simulink model "E55_1030"  (R2019b)
settings: Solver=FixedStepDiscrete  StartTime=0.0  StopTime=10  FixedStep=0.0005  RelTol=1e-3  EnableMultiTasking=on
InitFcn:
  | ecucoder_canfd
  | load('DATA_Plimit.mat')
  | a=0.775;
  | b=0.775;
  | kf=-50000;
  | kr=-50000;
  | m=226+75;
  | Iz=100;
  | u=0.85;
  | g=9.8;
  | L=a+b;
  | xi=0.1;
  | r=0.226;
  | Lw=1.171;
  | Tm=21;
  | i=15.9;
  | Jw=0.504;
  | Pmax=20000;
  | mw=19.3;
  | mb=148.9+75;
  | hg=0.280;
model workspace (MAT data in the model file):
  Initial_Steer_Position = 0
values from neighbouring files (symbols this model uses):
  SOC = [2.5 5 7.5 10 20 30 40 50 60 70 80 90 ... (14 elements, 14x1)]    [DATA_Plimit.mat]
  SOC_Discharge = [2.04592350211 2.57821618825 3.10671863859 3.63118835861 4.15200192786 4.66837694959 5.18149950051 5.69046162564 6.19532286188 6.696400261 7.19347596839 7.68712157998 ... (473 elements, 1x473)]    [DATA_Plimit.mat]
  VOLTAGE = [459.1488 476.0844 485.9448 487.344 492.822 498.8016 503.382 509.1108 518.8128 531.2472 544.5132 558.4656 ... (14 elements, 14x1)]    [DATA_Plimit.mat]
undefined symbols (not defined in the file or in its folder): DiscIntNeverNeededParam, H, HALL10, HALL6, HALL7, HALL8, HALL9, HPWM1, HPWM3, I_AN05_5V, I_AN07_5V, I_AN08_5V, I_AN09_5V, I_AN10_5V, I_SW11_H, I_SW12_H, I_SW13_H, I_SW14_H, I_SW15_H, I_SW16_H, I_SW17_H, I_SW18_H, I_SW19_H, LS1A2, O_HS1A2, O_HS1A8
libraries: ec311lib x152, simulink x92, canmsglib x30, canfdmsglib x2
(part 6 of 6)

== system E55_1030/Function-Call Subsystem2/Triggered Subsystem/AMK_Setpoints_Motor3/AMK_TorqueLimitNegativ ==
  AMK_TorqueLimitNegativ : Inport
  AMK_TorqueLimitNegativABS : Abs
  AMK_TorqueLimitNegativCOV : DataTypeConversion  OutDataTypeStr=uint8
  AMK_TorqueLimitNegativCS : ArithShift  BitShiftNumber=-16
  AMK_TorqueLimitNegativConS : Constant  OutDataTypeStr=single
  AMK_TorqueLimitNegativCosR : Constant  Value=0  OutDataTypeStr=uint8
  AMK_TorqueLimitNegativROP : RelationalOperator  Operator=<  OutDataTypeStr=boolean  RndMeth=Nearest
  AMK_TorqueLimitNegativRon : Rounding  Operator=round
  AMK_TorqueLimitNegativSW : Switch  Criteria=u2 ~= 0
  AMK_TorqueLimitNegativ_1sat : Saturate  UpperLimit=65535  LowerLimit=0
  AMK_TorqueLimitNegativ_And : simulink/Logic and Bit Operations/Bitwise Operator  logicop=AND  UseBitMask=off  NumInputPorts=2  BitMask=bin2dec('11011001')  BitMaskRealWorld=Stored Integer
  AMK_TorqueLimitNegativ_And_C : Constant  Value=255  OutDataTypeStr=uint32
  AMK_TorqueLimitNegativ_Convert : DataTypeConversion  OutDataTypeStr=uint32
  AMK_TorqueLimitNegativ_D : Product  Inputs=*/
  AMK_TorqueLimitNegativ_D1 : Product  Inputs=*/
  AMK_TorqueLimitNegativ_F : Constant  Value=0.1  OutDataTypeStr=single
  AMK_TorqueLimitNegativ_L : simulink/Logic and Bit Operations/Bitwise Operator  logicop=AND  UseBitMask=on  BitMask=65535  BitMaskRealWorld=Stored Integer
  AMK_TorqueLimitNegativ_O : Constant  Value=0  OutDataTypeStr=single
  AMK_TorqueLimitNegativ_S : ArithShift
  AMK_TorqueLimitNegativ_sat : Saturate  UpperLimit=0  LowerLimit=-100
  AMK_TorqueLimitNegativ_st : Sum  Inputs=+-
  AMK_TorqueLimitNegativoutput8_C : Constant  Value=256
  AMK_TorqueLimitNegativsubcon : Sum  Inputs=+-
  BitCov : DataTypeConversion  OutDataTypeStr=uint8
  Constant{1..6} (6 alike) : Constant  Value=0  OutDataTypeStr=uint8  SampleTime=-1
  output1 : Outport
  output2 : Outport  Port=2
  output3 : Outport  Port=3
  output4 : Outport  Port=4
  output5 : Outport  Port=5
  output6 : Outport  Port=6
  output7 : Outport  Port=7
  output8 : Outport  Port=8
  wires:
  Constant6/1 -> output6/1
  Constant5/1 -> output5/1
  Constant4/1 -> output4/1
  Constant3/1 -> output3/1
  Constant2/1 -> output2/1
  Constant1/1 -> output1/1
  BitCov/1 -> output7/1
  AMK_TorqueLimitNegativ_And/1 -> BitCov/1
  AMK_TorqueLimitNegativ_And_C/1 -> AMK_TorqueLimitNegativ_And/2
  AMK_TorqueLimitNegativCOV/1 -> output8/1
  AMK_TorqueLimitNegativ_D1/1 -> AMK_TorqueLimitNegativCOV/1
  AMK_TorqueLimitNegativoutput8_C/1 -> AMK_TorqueLimitNegativ_D1/2
  AMK_TorqueLimitNegativ_L/1 -> AMK_TorqueLimitNegativ_And/1, AMK_TorqueLimitNegativ_D1/1
  AMK_TorqueLimitNegativ_Convert/1 -> AMK_TorqueLimitNegativ_L/1
  AMK_TorqueLimitNegativ_1sat/1 -> AMK_TorqueLimitNegativ_Convert/1
  AMK_TorqueLimitNegativ_S/1 -> AMK_TorqueLimitNegativ_1sat/1
  AMK_TorqueLimitNegativSW/1 -> AMK_TorqueLimitNegativ_S/1
  AMK_TorqueLimitNegativROP/1 -> AMK_TorqueLimitNegativSW/2
  AMK_TorqueLimitNegativsubcon/1 -> AMK_TorqueLimitNegativSW/1
  AMK_TorqueLimitNegativABS/1 -> AMK_TorqueLimitNegativsubcon/2
  AMK_TorqueLimitNegativCS/1 -> AMK_TorqueLimitNegativsubcon/1
  AMK_TorqueLimitNegativConS/1 -> AMK_TorqueLimitNegativCS/1
  AMK_TorqueLimitNegativCosR/1 -> AMK_TorqueLimitNegativROP/2
  AMK_TorqueLimitNegativRon/1 -> AMK_TorqueLimitNegativSW/3, AMK_TorqueLimitNegativABS/1, AMK_TorqueLimitNegativROP/1
  AMK_TorqueLimitNegativ_D/1 -> AMK_TorqueLimitNegativRon/1
  AMK_TorqueLimitNegativ_F/1 -> AMK_TorqueLimitNegativ_D/2
  AMK_TorqueLimitNegativ_st/1 -> AMK_TorqueLimitNegativ_D/1
  AMK_TorqueLimitNegativ_O/1 -> AMK_TorqueLimitNegativ_st/2
  AMK_TorqueLimitNegativ_sat/1 -> AMK_TorqueLimitNegativ_st/1
  AMK_TorqueLimitNegativ/1 -> AMK_TorqueLimitNegativ_sat/1

== system E55_1030/Function-Call Subsystem2/Triggered Subsystem/AMK_Setpoints_Motor3/AMK_TorqueLimitPositiv ==
  AMK_TorqueLimitPositiv : Inport
  AMK_TorqueLimitPositivABS : Abs
  AMK_TorqueLimitPositivCOV : DataTypeConversion  OutDataTypeStr=uint8
  AMK_TorqueLimitPositivCS : ArithShift  BitShiftNumber=-16
  AMK_TorqueLimitPositivConS : Constant  OutDataTypeStr=single
  AMK_TorqueLimitPositivCosR : Constant  Value=0  OutDataTypeStr=uint8
  AMK_TorqueLimitPositivROP : RelationalOperator  Operator=<  OutDataTypeStr=boolean  RndMeth=Nearest
  AMK_TorqueLimitPositivRon : Rounding  Operator=round
  AMK_TorqueLimitPositivSW : Switch  Criteria=u2 ~= 0
  AMK_TorqueLimitPositiv_1sat : Saturate  UpperLimit=65535  LowerLimit=0
  AMK_TorqueLimitPositiv_And : simulink/Logic and Bit Operations/Bitwise Operator  logicop=AND  UseBitMask=off  NumInputPorts=2  BitMask=bin2dec('11011001')  BitMaskRealWorld=Stored Integer
  AMK_TorqueLimitPositiv_And_C : Constant  Value=255  OutDataTypeStr=uint32
  AMK_TorqueLimitPositiv_Convert : DataTypeConversion  OutDataTypeStr=uint32
  AMK_TorqueLimitPositiv_D : Product  Inputs=*/
  AMK_TorqueLimitPositiv_D1 : Product  Inputs=*/
  AMK_TorqueLimitPositiv_F : Constant  Value=0.1  OutDataTypeStr=single
  AMK_TorqueLimitPositiv_L : simulink/Logic and Bit Operations/Bitwise Operator  logicop=AND  UseBitMask=on  BitMask=65535  BitMaskRealWorld=Stored Integer
  AMK_TorqueLimitPositiv_O : Constant  Value=0  OutDataTypeStr=single
  AMK_TorqueLimitPositiv_S : ArithShift
  AMK_TorqueLimitPositiv_sat : Saturate  UpperLimit=100  LowerLimit=0
  AMK_TorqueLimitPositiv_st : Sum  Inputs=+-
  AMK_TorqueLimitPositivoutput6_C : Constant  Value=256
  AMK_TorqueLimitPositivsubcon : Sum  Inputs=+-
  BitCov : DataTypeConversion  OutDataTypeStr=uint8
  Constant{1..4,7..8} (6 alike) : Constant  Value=0  OutDataTypeStr=uint8  SampleTime=-1
  output1 : Outport
  output2 : Outport  Port=2
  output3 : Outport  Port=3
  output4 : Outport  Port=4
  output5 : Outport  Port=5
  output6 : Outport  Port=6
  output7 : Outport  Port=7
  output8 : Outport  Port=8
  wires:
  Constant8/1 -> output8/1
  Constant7/1 -> output7/1
  Constant4/1 -> output4/1
  Constant3/1 -> output3/1
  Constant2/1 -> output2/1
  Constant1/1 -> output1/1
  BitCov/1 -> output5/1
  AMK_TorqueLimitPositiv_And/1 -> BitCov/1
  AMK_TorqueLimitPositiv_And_C/1 -> AMK_TorqueLimitPositiv_And/2
  AMK_TorqueLimitPositivCOV/1 -> output6/1
  AMK_TorqueLimitPositiv_D1/1 -> AMK_TorqueLimitPositivCOV/1
  AMK_TorqueLimitPositivoutput6_C/1 -> AMK_TorqueLimitPositiv_D1/2
  AMK_TorqueLimitPositiv_L/1 -> AMK_TorqueLimitPositiv_And/1, AMK_TorqueLimitPositiv_D1/1
  AMK_TorqueLimitPositiv_Convert/1 -> AMK_TorqueLimitPositiv_L/1
  AMK_TorqueLimitPositiv_1sat/1 -> AMK_TorqueLimitPositiv_Convert/1
  AMK_TorqueLimitPositiv_S/1 -> AMK_TorqueLimitPositiv_1sat/1
  AMK_TorqueLimitPositivSW/1 -> AMK_TorqueLimitPositiv_S/1
  AMK_TorqueLimitPositivROP/1 -> AMK_TorqueLimitPositivSW/2
  AMK_TorqueLimitPositivsubcon/1 -> AMK_TorqueLimitPositivSW/1
  AMK_TorqueLimitPositivABS/1 -> AMK_TorqueLimitPositivsubcon/2
  AMK_TorqueLimitPositivCS/1 -> AMK_TorqueLimitPositivsubcon/1
  AMK_TorqueLimitPositivConS/1 -> AMK_TorqueLimitPositivCS/1
  AMK_TorqueLimitPositivCosR/1 -> AMK_TorqueLimitPositivROP/2
  AMK_TorqueLimitPositivRon/1 -> AMK_TorqueLimitPositivSW/3, AMK_TorqueLimitPositivABS/1, AMK_TorqueLimitPositivROP/1
  AMK_TorqueLimitPositiv_D/1 -> AMK_TorqueLimitPositivRon/1
  AMK_TorqueLimitPositiv_F/1 -> AMK_TorqueLimitPositiv_D/2
  AMK_TorqueLimitPositiv_st/1 -> AMK_TorqueLimitPositiv_D/1
  AMK_TorqueLimitPositiv_O/1 -> AMK_TorqueLimitPositiv_st/2
  AMK_TorqueLimitPositiv_sat/1 -> AMK_TorqueLimitPositiv_st/1
  AMK_TorqueLimitPositiv/1 -> AMK_TorqueLimitPositiv_sat/1

== system E55_1030/Function-Call Subsystem2/Triggered Subsystem/AMK_Setpoints_Motor4/AMK_Control ==
  AMK_Control : Inport
  AMK_ControlCOV : DataTypeConversion  OutDataTypeStr=uint8
  AMK_ControlRon : Rounding  Operator=round
  AMK_Control_1sat : Saturate  UpperLimit=65535  LowerLimit=0
  AMK_Control_And : simulink/Logic and Bit Operations/Bitwise Operator  logicop=AND  UseBitMask=off  NumInputPorts=2  BitMask=bin2dec('11011001')  BitMaskRealWorld=Stored Integer
  AMK_Control_And_C : Constant  Value=255  OutDataTypeStr=uint32
  AMK_Control_Convert : DataTypeConversion  OutDataTypeStr=uint32
  AMK_Control_D : Product  Inputs=*/
  AMK_Control_D1 : Product  Inputs=*/
  AMK_Control_F : Constant  OutDataTypeStr=single
  AMK_Control_L : simulink/Logic and Bit Operations/Bitwise Operator  logicop=AND  UseBitMask=on  BitMask=65535  BitMaskRealWorld=Stored Integer
  AMK_Control_O : Constant  Value=0  OutDataTypeStr=single
  AMK_Control_S : ArithShift
  AMK_Control_sat : Saturate  UpperLimit=65535  LowerLimit=0
  AMK_Control_st : Sum  Inputs=+-
  AMK_Controloutput2_C : Constant  Value=256
  BitCov : DataTypeConversion  OutDataTypeStr=uint8
  Constant{3..8} (6 alike) : Constant  Value=0  OutDataTypeStr=uint8  SampleTime=-1
  output1 : Outport
  output2 : Outport  Port=2
  output3 : Outport  Port=3
  output4 : Outport  Port=4
  output5 : Outport  Port=5
  output6 : Outport  Port=6
  output7 : Outport  Port=7
  output8 : Outport  Port=8
  wires:
  AMK_Control/1 -> AMK_Control_sat/1
  AMK_Control_sat/1 -> AMK_Control_st/1
  AMK_Control_O/1 -> AMK_Control_st/2
  AMK_Control_st/1 -> AMK_Control_D/1
  AMK_Control_F/1 -> AMK_Control_D/2
  AMK_Control_D/1 -> AMK_ControlRon/1
  AMK_ControlRon/1 -> AMK_Control_S/1
  AMK_Control_S/1 -> AMK_Control_1sat/1
  AMK_Control_1sat/1 -> AMK_Control_Convert/1
  AMK_Control_Convert/1 -> AMK_Control_L/1
  AMK_Control_L/1 -> AMK_Control_D1/1, AMK_Control_And/1
  AMK_Controloutput2_C/1 -> AMK_Control_D1/2
  AMK_Control_D1/1 -> AMK_ControlCOV/1
  AMK_ControlCOV/1 -> output2/1
  AMK_Control_And_C/1 -> AMK_Control_And/2
  AMK_Control_And/1 -> BitCov/1
  BitCov/1 -> output1/1
  Constant3/1 -> output3/1
  Constant4/1 -> output4/1
  Constant5/1 -> output5/1
  Constant6/1 -> output6/1
  Constant7/1 -> output7/1
  Constant8/1 -> output8/1

== system E55_1030/Function-Call Subsystem2/Triggered Subsystem/AMK_Setpoints_Motor4/AMK_TargetVelocity ==
  AMK_TargetVelocity : Inport
  AMK_TargetVelocityABS : Abs
  AMK_TargetVelocityCOV : DataTypeConversion  OutDataTypeStr=uint8
  AMK_TargetVelocityCS : ArithShift  BitShiftNumber=-16
  AMK_TargetVelocityConS : Constant  OutDataTypeStr=single
  AMK_TargetVelocityCosR : Constant  Value=0  OutDataTypeStr=uint8
  AMK_TargetVelocityROP : RelationalOperator  Operator=<  OutDataTypeStr=boolean  RndMeth=Nearest
  AMK_TargetVelocityRon : Rounding  Operator=round
  AMK_TargetVelocitySW : Switch  Criteria=u2 ~= 0
  AMK_TargetVelocity_1sat : Saturate  UpperLimit=65535  LowerLimit=0
  AMK_TargetVelocity_And : simulink/Logic and Bit Operations/Bitwise Operator  logicop=AND  UseBitMask=off  NumInputPorts=2  BitMask=bin2dec('11011001')  BitMaskRealWorld=Stored Integer
  AMK_TargetVelocity_And_C : Constant  Value=255  OutDataTypeStr=uint32
  AMK_TargetVelocity_Convert : DataTypeConversion  OutDataTypeStr=uint32
  AMK_TargetVelocity_D : Product  Inputs=*/
  AMK_TargetVelocity_D1 : Product  Inputs=*/
  AMK_TargetVelocity_F : Constant  OutDataTypeStr=single
  AMK_TargetVelocity_L : simulink/Logic and Bit Operations/Bitwise Operator  logicop=AND  UseBitMask=on  BitMask=65535  BitMaskRealWorld=Stored Integer
  AMK_TargetVelocity_O : Constant  Value=0  OutDataTypeStr=single
  AMK_TargetVelocity_S : ArithShift
  AMK_TargetVelocity_sat : Saturate  UpperLimit=32767  LowerLimit=-32768
  AMK_TargetVelocity_st : Sum  Inputs=+-
  AMK_TargetVelocityoutput4_C : Constant  Value=256
  AMK_TargetVelocitysubcon : Sum  Inputs=+-
  BitCov : DataTypeConversion  OutDataTypeStr=uint8
  Constant{1..2,5..8} (6 alike) : Constant  Value=0  OutDataTypeStr=uint8  SampleTime=-1
  output1 : Outport
  output2 : Outport  Port=2
  output3 : Outport  Port=3
  output4 : Outport  Port=4
  output5 : Outport  Port=5
  output6 : Outport  Port=6
  output7 : Outport  Port=7
  output8 : Outport  Port=8
  wires:
  AMK_TargetVelocity/1 -> AMK_TargetVelocity_sat/1
  AMK_TargetVelocity_sat/1 -> AMK_TargetVelocity_st/1
  AMK_TargetVelocity_O/1 -> AMK_TargetVelocity_st/2
  AMK_TargetVelocity_st/1 -> AMK_TargetVelocity_D/1
  AMK_TargetVelocity_F/1 -> AMK_TargetVelocity_D/2
  AMK_TargetVelocity_D/1 -> AMK_TargetVelocityRon/1
  AMK_TargetVelocityRon/1 -> AMK_TargetVelocityROP/1, AMK_TargetVelocityABS/1, AMK_TargetVelocitySW/3
  AMK_TargetVelocityCosR/1 -> AMK_TargetVelocityROP/2
  AMK_TargetVelocityConS/1 -> AMK_TargetVelocityCS/1
  AMK_TargetVelocityCS/1 -> AMK_TargetVelocitysubcon/1
  AMK_TargetVelocityABS/1 -> AMK_TargetVelocitysubcon/2
  AMK_TargetVelocitysubcon/1 -> AMK_TargetVelocitySW/1
  AMK_TargetVelocityROP/1 -> AMK_TargetVelocitySW/2
  AMK_TargetVelocitySW/1 -> AMK_TargetVelocity_S/1
  AMK_TargetVelocity_S/1 -> AMK_TargetVelocity_1sat/1
  AMK_TargetVelocity_1sat/1 -> AMK_TargetVelocity_Convert/1
  AMK_TargetVelocity_Convert/1 -> AMK_TargetVelocity_L/1
  AMK_TargetVelocity_L/1 -> AMK_TargetVelocity_D1/1, AMK_TargetVelocity_And/1
  AMK_TargetVelocityoutput4_C/1 -> AMK_TargetVelocity_D1/2
  AMK_TargetVelocity_D1/1 -> AMK_TargetVelocityCOV/1
  AMK_TargetVelocityCOV/1 -> output4/1
  AMK_TargetVelocity_And_C/1 -> AMK_TargetVelocity_And/2
  AMK_TargetVelocity_And/1 -> BitCov/1
  BitCov/1 -> output3/1
  Constant1/1 -> output1/1
  Constant2/1 -> output2/1
  Constant5/1 -> output5/1
  Constant6/1 -> output6/1
  Constant7/1 -> output7/1
  Constant8/1 -> output8/1

== system E55_1030/Function-Call Subsystem2/Triggered Subsystem/AMK_Setpoints_Motor4/AMK_TorqueLimitNegativ ==
  AMK_TorqueLimitNegativ : Inport
  AMK_TorqueLimitNegativABS : Abs
  AMK_TorqueLimitNegativCOV : DataTypeConversion  OutDataTypeStr=uint8
  AMK_TorqueLimitNegativCS : ArithShift  BitShiftNumber=-16
  AMK_TorqueLimitNegativConS : Constant  OutDataTypeStr=single
  AMK_TorqueLimitNegativCosR : Constant  Value=0  OutDataTypeStr=uint8
  AMK_TorqueLimitNegativROP : RelationalOperator  Operator=<  OutDataTypeStr=boolean  RndMeth=Nearest
  AMK_TorqueLimitNegativRon : Rounding  Operator=round
  AMK_TorqueLimitNegativSW : Switch  Criteria=u2 ~= 0
  AMK_TorqueLimitNegativ_1sat : Saturate  UpperLimit=65535  LowerLimit=0
  AMK_TorqueLimitNegativ_And : simulink/Logic and Bit Operations/Bitwise Operator  logicop=AND  UseBitMask=off  NumInputPorts=2  BitMask=bin2dec('11011001')  BitMaskRealWorld=Stored Integer
  AMK_TorqueLimitNegativ_And_C : Constant  Value=255  OutDataTypeStr=uint32
  AMK_TorqueLimitNegativ_Convert : DataTypeConversion  OutDataTypeStr=uint32
  AMK_TorqueLimitNegativ_D : Product  Inputs=*/
  AMK_TorqueLimitNegativ_D1 : Product  Inputs=*/
  AMK_TorqueLimitNegativ_F : Constant  Value=0.1  OutDataTypeStr=single
  AMK_TorqueLimitNegativ_L : simulink/Logic and Bit Operations/Bitwise Operator  logicop=AND  UseBitMask=on  BitMask=65535  BitMaskRealWorld=Stored Integer
  AMK_TorqueLimitNegativ_O : Constant  Value=0  OutDataTypeStr=single
  AMK_TorqueLimitNegativ_S : ArithShift
  AMK_TorqueLimitNegativ_sat : Saturate  UpperLimit=0  LowerLimit=-100
  AMK_TorqueLimitNegativ_st : Sum  Inputs=+-
  AMK_TorqueLimitNegativoutput8_C : Constant  Value=256
  AMK_TorqueLimitNegativsubcon : Sum  Inputs=+-
  BitCov : DataTypeConversion  OutDataTypeStr=uint8
  Constant{1..6} (6 alike) : Constant  Value=0  OutDataTypeStr=uint8  SampleTime=-1
  output1 : Outport
  output2 : Outport  Port=2
  output3 : Outport  Port=3
  output4 : Outport  Port=4
  output5 : Outport  Port=5
  output6 : Outport  Port=6
  output7 : Outport  Port=7
  output8 : Outport  Port=8
  wires:
  AMK_TorqueLimitNegativ/1 -> AMK_TorqueLimitNegativ_sat/1
  AMK_TorqueLimitNegativ_sat/1 -> AMK_TorqueLimitNegativ_st/1
  AMK_TorqueLimitNegativ_O/1 -> AMK_TorqueLimitNegativ_st/2
  AMK_TorqueLimitNegativ_st/1 -> AMK_TorqueLimitNegativ_D/1
  AMK_TorqueLimitNegativ_F/1 -> AMK_TorqueLimitNegativ_D/2
  AMK_TorqueLimitNegativ_D/1 -> AMK_TorqueLimitNegativRon/1
  AMK_TorqueLimitNegativRon/1 -> AMK_TorqueLimitNegativROP/1, AMK_TorqueLimitNegativABS/1, AMK_TorqueLimitNegativSW/3
  AMK_TorqueLimitNegativCosR/1 -> AMK_TorqueLimitNegativROP/2
  AMK_TorqueLimitNegativConS/1 -> AMK_TorqueLimitNegativCS/1
  AMK_TorqueLimitNegativCS/1 -> AMK_TorqueLimitNegativsubcon/1
  AMK_TorqueLimitNegativABS/1 -> AMK_TorqueLimitNegativsubcon/2
  AMK_TorqueLimitNegativsubcon/1 -> AMK_TorqueLimitNegativSW/1
  AMK_TorqueLimitNegativROP/1 -> AMK_TorqueLimitNegativSW/2
  AMK_TorqueLimitNegativSW/1 -> AMK_TorqueLimitNegativ_S/1
  AMK_TorqueLimitNegativ_S/1 -> AMK_TorqueLimitNegativ_1sat/1
  AMK_TorqueLimitNegativ_1sat/1 -> AMK_TorqueLimitNegativ_Convert/1
  AMK_TorqueLimitNegativ_Convert/1 -> AMK_TorqueLimitNegativ_L/1
  AMK_TorqueLimitNegativ_L/1 -> AMK_TorqueLimitNegativ_D1/1, AMK_TorqueLimitNegativ_And/1
  AMK_TorqueLimitNegativoutput8_C/1 -> AMK_TorqueLimitNegativ_D1/2
  AMK_TorqueLimitNegativ_D1/1 -> AMK_TorqueLimitNegativCOV/1
  AMK_TorqueLimitNegativCOV/1 -> output8/1
  AMK_TorqueLimitNegativ_And_C/1 -> AMK_TorqueLimitNegativ_And/2
  AMK_TorqueLimitNegativ_And/1 -> BitCov/1
  BitCov/1 -> output7/1
  Constant1/1 -> output1/1
  Constant2/1 -> output2/1
  Constant3/1 -> output3/1
  Constant4/1 -> output4/1
  Constant5/1 -> output5/1
  Constant6/1 -> output6/1

== system E55_1030/Function-Call Subsystem2/Triggered Subsystem/AMK_Setpoints_Motor4/AMK_TorqueLimitPositiv ==
  AMK_TorqueLimitPositiv : Inport
  AMK_TorqueLimitPositivABS : Abs
  AMK_TorqueLimitPositivCOV : DataTypeConversion  OutDataTypeStr=uint8
  AMK_TorqueLimitPositivCS : ArithShift  BitShiftNumber=-16
  AMK_TorqueLimitPositivConS : Constant  OutDataTypeStr=single
  AMK_TorqueLimitPositivCosR : Constant  Value=0  OutDataTypeStr=uint8
  AMK_TorqueLimitPositivROP : RelationalOperator  Operator=<  OutDataTypeStr=boolean  RndMeth=Nearest
  AMK_TorqueLimitPositivRon : Rounding  Operator=round
  AMK_TorqueLimitPositivSW : Switch  Criteria=u2 ~= 0
  AMK_TorqueLimitPositiv_1sat : Saturate  UpperLimit=65535  LowerLimit=0
  AMK_TorqueLimitPositiv_And : simulink/Logic and Bit Operations/Bitwise Operator  logicop=AND  UseBitMask=off  NumInputPorts=2  BitMask=bin2dec('11011001')  BitMaskRealWorld=Stored Integer
  AMK_TorqueLimitPositiv_And_C : Constant  Value=255  OutDataTypeStr=uint32
  AMK_TorqueLimitPositiv_Convert : DataTypeConversion  OutDataTypeStr=uint32
  AMK_TorqueLimitPositiv_D : Product  Inputs=*/
  AMK_TorqueLimitPositiv_D1 : Product  Inputs=*/
  AMK_TorqueLimitPositiv_F : Constant  Value=0.1  OutDataTypeStr=single
  AMK_TorqueLimitPositiv_L : simulink/Logic and Bit Operations/Bitwise Operator  logicop=AND  UseBitMask=on  BitMask=65535  BitMaskRealWorld=Stored Integer
  AMK_TorqueLimitPositiv_O : Constant  Value=0  OutDataTypeStr=single
  AMK_TorqueLimitPositiv_S : ArithShift
  AMK_TorqueLimitPositiv_sat : Saturate  UpperLimit=100  LowerLimit=0
  AMK_TorqueLimitPositiv_st : Sum  Inputs=+-
  AMK_TorqueLimitPositivoutput6_C : Constant  Value=256
  AMK_TorqueLimitPositivsubcon : Sum  Inputs=+-
  BitCov : DataTypeConversion  OutDataTypeStr=uint8
  Constant{1..4,7..8} (6 alike) : Constant  Value=0  OutDataTypeStr=uint8  SampleTime=-1
  output1 : Outport
  output2 : Outport  Port=2
  output3 : Outport  Port=3
  output4 : Outport  Port=4
  output5 : Outport  Port=5
  output6 : Outport  Port=6
  output7 : Outport  Port=7
  output8 : Outport  Port=8
  wires:
  AMK_TorqueLimitPositiv/1 -> AMK_TorqueLimitPositiv_sat/1
  AMK_TorqueLimitPositiv_sat/1 -> AMK_TorqueLimitPositiv_st/1
  AMK_TorqueLimitPositiv_O/1 -> AMK_TorqueLimitPositiv_st/2
  AMK_TorqueLimitPositiv_st/1 -> AMK_TorqueLimitPositiv_D/1
  AMK_TorqueLimitPositiv_F/1 -> AMK_TorqueLimitPositiv_D/2
  AMK_TorqueLimitPositiv_D/1 -> AMK_TorqueLimitPositivRon/1
  AMK_TorqueLimitPositivRon/1 -> AMK_TorqueLimitPositivROP/1, AMK_TorqueLimitPositivABS/1, AMK_TorqueLimitPositivSW/3
  AMK_TorqueLimitPositivCosR/1 -> AMK_TorqueLimitPositivROP/2
  AMK_TorqueLimitPositivConS/1 -> AMK_TorqueLimitPositivCS/1
  AMK_TorqueLimitPositivCS/1 -> AMK_TorqueLimitPositivsubcon/1
  AMK_TorqueLimitPositivABS/1 -> AMK_TorqueLimitPositivsubcon/2
  AMK_TorqueLimitPositivsubcon/1 -> AMK_TorqueLimitPositivSW/1
  AMK_TorqueLimitPositivROP/1 -> AMK_TorqueLimitPositivSW/2
  AMK_TorqueLimitPositivSW/1 -> AMK_TorqueLimitPositiv_S/1
  AMK_TorqueLimitPositiv_S/1 -> AMK_TorqueLimitPositiv_1sat/1
  AMK_TorqueLimitPositiv_1sat/1 -> AMK_TorqueLimitPositiv_Convert/1
  AMK_TorqueLimitPositiv_Convert/1 -> AMK_TorqueLimitPositiv_L/1
  AMK_TorqueLimitPositiv_L/1 -> AMK_TorqueLimitPositiv_D1/1, AMK_TorqueLimitPositiv_And/1
  AMK_TorqueLimitPositivoutput6_C/1 -> AMK_TorqueLimitPositiv_D1/2
  AMK_TorqueLimitPositiv_D1/1 -> AMK_TorqueLimitPositivCOV/1
  AMK_TorqueLimitPositivCOV/1 -> output6/1
  AMK_TorqueLimitPositiv_And_C/1 -> AMK_TorqueLimitPositiv_And/2
  AMK_TorqueLimitPositiv_And/1 -> BitCov/1
  BitCov/1 -> output5/1
  Constant1/1 -> output1/1
  Constant2/1 -> output2/1
  Constant3/1 -> output3/1
  Constant4/1 -> output4/1
  Constant7/1 -> output7/1
  Constant8/1 -> output8/1

== stateflow chart E55_1030/Function-Call Subsystem2/StateChange1 ==
  state S1
    du:flag_regen=0;
  state S2
    du:flag_regen=1;
  (default) -> S1
  S1 -> S2 : [run_flag==3&&brake_pressure_r>0.9&&acc<2.5]
  S2 -> S1 : [run_flag==3&&brake_pressure_r<0.85&&acc<1]
  data: acc input; flag_regen output; brake_pressure_r input; run_flag input

== stateflow chart E55_1030/Function-Call Subsystem2/StateChange3 ==
  state S3
    du:one_motor=1
  state S1
    du:one_motor=1
  state S2
    du:one_motor=0
  (default) -> S3
  S3 -> S1 : [runflag==3]
  S1 -> S2 : [after(2,sec) && start_input==1&&reset_input==1]
      | {one_motor=0}
  S2 -> S1 [order 2] : [after(2,sec)&&start_input==1&&reset_input==1]{one_motor=1}
  S2 -> S3 [order 1] : [runflag~=3]{one_motor=1}
  data: runflag input; one_motor output; start_input input; flag local double; reset_input input

== matlab function E55_1030/Function-Call Subsystem2/MATLAB Function ==
  data: input_data input; avg output
function avg = movingAverage(input_data)
    % 参数定义
    window_size = 100; % 滑动窗口大小

    % 初始化变量
    persistent data_buffer;
    persistent sum_buffer;
    if isempty(data_buffer)
        data_buffer = zeros(1, window_size);
        sum_buffer = 0;
    end

    % 更新缓冲区
    sum_buffer = sum_buffer - data_buffer(1) + input_data;
    data_buffer = circshift(data_buffer, [0, -1]);
    data_buffer(end) = input_data;

    % 计算平均值
    avg = sum_buffer / window_size;
end

== stateflow chart E55_1030/Function-Call Subsystem2/StateChange2 ==
  state S [parallel]
    settings: executionOrder=2
    state S2
      du:runflag=2;
      readyLED_output=false;
    state S1
      du:runflag=1;
      readyLED_output=false;
    state S3
      du:runflag=3;
      readyLED_output=true;
      zero_count=0;
    state S4
      du:zero_count=zero_count+1;
    S1 -> S2 : [acc_flag==1 ...
        | &&safe_input==1 ...
        | &&precharge_input>0]
    S2 -> S1 [order 2] : [safe_input == 0]
    S4 -> S1 [order 2] : [zero_count == 100]
    S2 -> S3 [order 1] : [start_input>0&&break_output>5&&break_output<99&&BMS_state==2]
    S4 -> S3 [order 1] : [safe_input==1]
    S3 -> S4 : [safe_input==0]
  state B [parallel]
    settings: executionOrder=1
    state B1
      du:beep=0;
    state B2
      du:beep=1;
    state B3
      du:beep=0;
    (default) -> B1
    B1 -> B2 : [in(S.S3)]
    B2 -> B3 : [after(1,sec)]
    B3 -> B1 : [in(S.S1)]
  (default) -> S1
  data: acc_flag input; safe_input input; precharge_input input; start_input input; runflag output double; readyLED_output output boolean; beep output; break_output input; zero_count local [0..10000] =0; BMS_state input

== matlab function E55_1030/Function-Call Subsystem2/MATLAB Function16 ==
  data: input_data input; avg output
function avg = movingAverage(input_data)
    % 参数定义
    window_size = 200; % 滑动窗口大小

    % 初始化变量
    persistent data_buffer;
    persistent sum_buffer;
    if isempty(data_buffer)
        data_buffer = zeros(1, window_size);
        sum_buffer = 0;
    end

    % 更新缓冲区
    sum_buffer = sum_buffer - data_buffer(1) + input_data;
    data_buffer = circshift(data_buffer, [0, -1]);
    data_buffer(end) = input_data;

    % 计算平均值
    avg = sum_buffer / window_size;
end

== matlab function E55_1030/Function-Call Subsystem2/MATLAB Function1 ==
  data: East_Speed input; Heading_Angle output; North_Speed input; Yaw_Angle input
function Heading_Angle = count_Heading_Angle(East_Speed, North_Speed, Yaw_Angle)
if(abs(East_Speed)<2 && abs(North_Speed)<2)
    Heading_Angle = Yaw_Angle;
else
    if(atan2(East_Speed, North_Speed)>=0)
        Heading_Angle = atan2(East_Speed, North_Speed) * 180 / pi;
    else
        Heading_Angle = atan2(East_Speed, North_Speed) * 180 / pi + 360;
    end
end

== matlab function E55_1030/Function-Call Subsystem2/MATLAB Function2 ==
  data: Yaw_Angle input; Acc_X output; Pitch_Angle input; Roll_Angle input; Acc_X_with_g input; Acc_Y_with_g input; Acc_Z_with_g input; Acc_Y output; Acc_Z output
function [Acc_X, Acc_Y, Acc_Z] = Transformation(Yaw_Angle, Pitch_Angle, Roll_Angle, Acc_X_with_g, Acc_Y_with_g, Acc_Z_with_g)
att = [Pitch_Angle;-1*Roll_Angle;Yaw_Angle];
gravity = [0;0;-9.8];
gravity_b = ch_eul2m(att)*gravity;
Acc_X = Acc_X_with_g - gravity_b(1);
Acc_Y = Acc_Y_with_g - gravity_b(2);
Acc_Z = Acc_Z_with_g - gravity_b(3);


function Cb2n_312 = ch_eul2m(att)
% 将欧拉角转换为姿态阵
% 复用严龚敏老师的a2mat
%
% Input: att  单位：rad
% 对于312(Z->X->Y)顺序，对应att = [pitch(绕X轴) roll(绕Y轴)  yaw(绕Z轴)]
% 对于321(Z->Y->X)顺序，对应att = [roll(绕X轴) pitch(绕Y轴)  yaw(绕Z轴)]
% Outputs: 
% Cb2n_312:  312欧拉角顺序下转换后的Cb2n
% Cb2n_321:  321欧拉角顺序下转换后的Cb2n

    s = sin(att); c = cos(att);
    si = s(1); sj = s(2); sk = s(3); 
    ci = c(1); cj = c(2); ck = c(3);
    Cb2n_312 = [ cj*ck-si*sj*sk, -ci*sk,  sj*ck+si*cj*sk;
                 cj*sk+si*sj*ck,  ci*ck,  sj*sk-si*cj*ck;
                -ci*sj,           si,     ci*cj          ];

== matlab function E55_1030/Function-Call Subsystem2/MATLAB Function3 ==
  data: delta_angle input; Yaw_Rate output
function Yaw_Rate = derivative(delta_angle)
if(delta_angle<0)
    if(abs(delta_angle)>180)
        delta_angle_cor = delta_angle + 360;
    else
        delta_angle_cor = delta_angle;
    end
else
    if(abs(delta_angle)>180)
        delta_angle_cor = delta_angle - 360;
    else
        delta_angle_cor = delta_angle;
    end
end
Yaw_Rate = delta_angle_cor/0.1;

== matlab function E55_1030/Function-Call Subsystem2/MATLAB Function4 ==
  data: Heading_Angle input; Side_Slip_Angle output; Yaw_Angle input
function Side_Slip_Angle = count_Side_Slip_Angle(Heading_Angle, Yaw_Angle)
persistent data_buffer;
if isempty(data_buffer)
    data_buffer = 0; % 初始化上一个时刻的值为0或者适当的初始值
end

Side_Slip_Angle = Yaw_Angle - Heading_Angle;
if(Side_Slip_Angle>180)
    Side_Slip_Angle = Side_Slip_Angle - 360;
elseif(Side_Slip_Angle<-180)
    Side_Slip_Angle = Side_Slip_Angle + 360;
end

if Side_Slip_Angle>10||Side_Slip_Angle<-10
    Side_Slip_Angle = data_buffer;
else
    data_buffer = Side_Slip_Angle;
end

== matlab function E55_1030/Function-Call Subsystem2/MATLAB Function5 ==
  data: Torque_req input; Torque output; Mz input; steer_angle input; yaw_rate input; yaw_rate_d input; break_state input; T_max input; factor_F input; factor_R input
function Torque = Torque_Distribution(Torque_req,Mz,steer_angle,yaw_rate,yaw_rate_d,break_state,T_max, factor_F, factor_R)
    r = 0.2286;%Tire radius
    Lw = 1.171;%Track width
    e = yaw_rate - yaw_rate_d;
    delta_T = Mz*r*saturation(e,0.05)*saturation(steer_angle,1)*Throttle_Zero_Zone(Torque_req)/Lw;
    i = 15.9;
    
    if(break_state>5 && Torque_req<0.05)
        T_fr = 0;
        T_fl = 0;
        T_rr = 0;
        T_rl = 0;
    else
        if(steer_angle<=0)%left is greater
            if(Torque_req*max(T_max)*i + delta_T>max(T_max)*i)
                T_fr = T_max(1)*i - 2*delta_T;
                T_fl = T_max(2)*i;
                T_rr = T_max(3)*i - 2*delta_T;
                T_rl = T_max(4)*i;
            elseif(Torque_req*min(T_max)*i - delta_T<0)
                T_fr = 0;
                T_fl = 2*delta_T;
                T_rr = 0;
                T_rl = 2*delta_T;
            else
                T_fr = Torque_req*T_max(1)*i*factor_F - delta_T;
                T_fl = Torque_req*T_max(2)*i*factor_F + delta_T;
                T_rr = Torque_req*T_max(3)*i*factor_R - delta_T;
                T_rl = Torque_req*T_max(4)*i*factor_R + delta_T;
            end
        else%right is greater
            if(Torque_req*max(T_max)*i + delta_T>max(T_max)*i)
                T_fr = T_max(1)*i;
                T_fl = T_max(2)*i - 2*delta_T;
                T_rr = T_max(3)*i;
                T_rl = T_max(4)*i - 2*delta_T;
            elseif(Torque_req*min(T_max)*i - delta_T<0)
                T_fr = 2*delta_T;
                T_fl = 0;
                T_rr = 2*delta_T;
                T_rl = 0;
            else
                T_fr = Torque_req*T_max(1)*i*factor_F + delta_T;
                T_fl = Torque_req*T_max(2)*i*factor_F - delta_T;
                T_rr = Torque_req*T_max(3)*i*factor_R + delta_T;
                T_rl = Torque_req*T_max(4)*i*factor_R - delta_T;
            end
        end
    end
    Torque = [T_fl;T_fr;T_rl;T_rr];
    
function sat = saturation(in,delta)
    if(abs(in)>delta)
        sat = 1;
    else
        sat = abs(in)/delta;
    end
    
function output = Throttle_Zero_Zone(throttle)
    if(throttle<0.05)
        output = 10*throttle + 0.5;
    else
        output = 1;
    end

== matlab function E55_1030/Function-Call Subsystem2/MATLAB Function6 ==
  data: runflag input; TargetVelocity output; acc_flag input; start_input input; reset_state input; flag_regen input
function TargetVelocity = Set_TargetVelocity(runflag, acc_flag, start_input, reset_state, flag_regen)
if(runflag<3 || acc_flag==0 || reset_state || flag_regen)
    TargetVelocity = 0;
elseif(start_input==1)
    TargetVelocity = -5000;
else
    TargetVelocity = 20000;
end

== matlab function E55_1030/Function-Call Subsystem2/MATLAB Function7 ==
  data: acc1 input; acc_flag output; acc2 input
function acc_flag = count_acc_flag(acc1, acc2)
delta_acc = abs(acc1-acc2);
if(delta_acc<10)
    acc_flag = 1;
else
    acc_flag = 0;
end

== matlab function E55_1030/Function-Call Subsystem2/MATLAB Function8 ==
  data: break_input input; break_light output
function break_light = break_light_enable(break_input)
if(break_input>30)
    break_light = 1;
else
    break_light = 0;
end

== matlab function E55_1030/Function-Call Subsystem2/SMC_ASR/MATLAB Function ==
  data: Torque_input input; Torque_ASR output; T_max input
function Torque_ASR = Power_Limit(Torque_input, T_max)
Torque_ASR = [0,0,0,0];
for i=1:4
    if(Torque_input(i)>T_max(i))
        Torque_ASR(i) = T_max(i);
    elseif(Torque_input(i)<0)
        Torque_ASR(i) = 0;
    else
        Torque_ASR(i) = Torque_input(i);
    end
end

== matlab function E55_1030/Function-Call Subsystem2/MATLAB Function9 ==
  data: acc1_input input; acc_out output; acc2_input input
function acc_out = count_acc(acc1_input,acc2_input)
if(acc1_input<50 || acc2_input<50)
    acc_out = 0;
else
    acc_out = 1;
end

== matlab function E55_1030/Function-Call Subsystem2/MATLAB Function10 ==
  data: Yaw_Angle input; K3105G_flag output; Pitch_Angle input; Roll_Angle input
function K3105G_flag = is_K3015G_working(Yaw_Angle, Pitch_Angle, Roll_Angle)
if(Yaw_Angle == -360 && Pitch_Angle == -360 && Roll_Angle == -360)
    K3105G_flag = 0;
else
    K3105G_flag = 1;
end

== matlab function E55_1030/Function-Call Subsystem2/MATLAB Function11 ==
  data: East_Speed input; Velocity output; North_Speed input
function Velocity = count_velocity(East_Speed, North_Speed)
if(East_Speed == -100 && North_Speed == -100)
    Velocity = 0;
else
    Velocity = sqrt(East_Speed * East_Speed + North_Speed * North_Speed);
end

== matlab function E55_1030/Function-Call Subsystem2/驱动防滑使能/MATLAB Function ==
  data: wheel_speed input; s output; wheel_speed_d input
function s = count_slip_ratio(wheel_speed, wheel_speed_d)
s = zeros(4,1);
for i = 1:4
    if wheel_speed(i)<=100 && wheel_speed_d(i)<=100
        s(i) = 0;
    else
        s(i) = abs((wheel_speed(i) - wheel_speed_d(i))/wheel_speed(i));
    end
end

== stateflow chart E55_1030/Function-Call Subsystem2/StateChange4 ==
  state S2
    du:Algorithm_Enable=1
  state S1
    du:Algorithm_Enable=0
  state S3
    du:Algorithm_Enable=0
  (default) -> S3
  S3 -> S1 : [runflag==3]
  S1 -> S2 : [after(2,sec) && precharge_input==1&&reset_input==1]
  S2 -> S1 [order 2] : [after(2,sec)&&precharge_input==1&&reset_input==1]
  S2 -> S3 [order 1] : [runflag~=3]
  data: runflag input; Algorithm_Enable output; precharge_input input; flag local double; reset_input input

== matlab function E55_1030/Function-Call Subsystem2/MATLAB Function12 ==
  data: K3105G_flag input; flag output; Algorithm_Enable input; Runflag input
function flag = Enable(K3105G_flag, Algorithm_Enable, Runflag)
if(K3105G_flag == 1 && Runflag==3)
    flag = Algorithm_Enable;
else
    flag = 0;
end

== matlab function E55_1030/Function-Call Subsystem2/If Action Subsystem15/MATLAB Function ==
  data: Throttle input; factor_F output
function factor_F = fcn(Throttle)
if(Throttle<10)
    factor_F = 1;
elseif(Throttle<60)
    factor_F = 0.2+8/Throttle;
else
    factor_F = 2-100/Throttle;
end

== matlab function E55_1030/Function-Call Subsystem2/MATLAB Function13 ==
  data: Throttle input; factor_F output
function factor_F = fcn(Throttle)
if(Throttle<10)
    factor_F = 1;
elseif(Throttle<60)
    factor_F = 0.2+8/Throttle;
else
    factor_F = 2-100/Throttle;
end

== matlab function E55_1030/Function-Call Subsystem2/MATLAB Function14 ==
  data: Throttle input; factor_R output
function factor_R = fcn(Throttle)
if(Throttle<10)
    factor_R = 1;
elseif(Throttle<60)
    factor_R = 1.4 - 4/Throttle;
else
    factor_R = 0.5 + 50/Throttle;
end

== matlab function E55_1030/Function-Call Subsystem2/If Action Subsystem15/MATLAB Function14 ==
  data: Throttle input; factor_R output
function factor_R = fcn(Throttle)
if(Throttle<10)
    factor_R = 1;
elseif(Throttle<60)
    factor_R = 1.4 - 4/Throttle;
else
    factor_R = 0.5 + 50/Throttle;
end

== matlab function E55_1030/Function-Call Subsystem2/计算理想横摆角速度和质心侧偏角/MATLAB Function ==
  data: in input; Yaw_Rate_d output; Yaw_Rate input; K3105G_flag input; Velocity input
function Yaw_Rate_d = fcn(in, Yaw_Rate, K3105G_flag, Velocity)
if K3105G_flag == 0 || Velocity < 5/3.6
    Yaw_Rate_d = Yaw_Rate;
else
    Yaw_Rate_d = in;
end

== matlab function E55_1030/Function-Call Subsystem2/计算理想横摆角速度和质心侧偏角/MATLAB Function1 ==
  data: in input; Side_Slip_Angle_d output; Side_Slip_Angle input; K3105G_flag input; Velocity input
function Side_Slip_Angle_d = fcn(in, Side_Slip_Angle, K3105G_flag, Velocity)
if K3105G_flag == 0 || Velocity < 5/3.6
    Side_Slip_Angle_d = Side_Slip_Angle;
else
    Side_Slip_Angle_d = in;
end

== matlab function E55_1030/Function-Call Subsystem2/Subsystem17/MATLAB Function ==
  data: a1 input; Tx34 output; a2 input; b1 input; b2 input
function Tx34 = fcn(a1, a2, b1, b2)

Tx34=inv([a1,0;0,a2;])*[b1;b2;];

== matlab function E55_1030/Function-Call Subsystem2/Subsystem17/MATLAB Function1 ==
  data: Torque_input input; T_max input; Tx3 output; Tx4 output
function [Tx3,Tx4] = Power_Limit(Torque_input, T_max)

if(Torque_input(1)>T_max(3))
    Tx3 = T_max(3);
elseif(Torque_input(1)<0)
    Tx3 = 0;
else
    Tx3 = Torque_input(1);
end

if(Torque_input(2)>T_max(4))
    Tx4 = T_max(3);
elseif(Torque_input(2)<0)
    Tx4 = 0;
else
    Tx4 = Torque_input(2);
end

== matlab function E55_1030/Function-Call Subsystem2/Subsystem17/MATLAB Function2 ==
  data: Torque_input input; T_max input; Tx1 output
function Tx1 = Power_Limit(Torque_input, T_max)

if(Torque_input>T_max(1))
    Tx1 = T_max(1);
elseif(Torque_input<0)
    Tx1 = 0;
else
    Tx1 = Torque_input;
end

== matlab function E55_1030/Function-Call Subsystem2/Subsystem17/MATLAB Function3 ==
  data: T_max input; Torque_input input; Tx2 output
function Tx2 = Power_Limit(T_max, Torque_input)

if(Torque_input>T_max(2))
    Tx2 = T_max(2);
elseif(Torque_input<0)
    Tx2 = 0;
else
    Tx2 = Torque_input;
end

== stateflow chart E55_1030/Function-Call Subsystem2/StateChange5 ==
  state S3
    du:reset_state=0;
    reset_count=0;
  state S1
    du:reset_state=1;
    reset_count=0;
  state S4
    du:reset_count=reset_count+1
  state S5
    du:reset_state=0;
    reset_count=0;
  state S6
    du:reset_count=reset_count+1
  state S7
    du:reset_state=1;
    reset_count=0;
  (default) -> S3
  S3 -> S1 : [run_flag==2]
  S1 -> S4 : [run_flag==3]
  S4 -> S5 : [reset_count==30]
  S5 -> S7 : [reset_input==1]
  S7 -> S6 : [reset_input==0]
  S6 -> S7 [order 2] : [reset_input==1]
  S6 -> S5 [order 1] : [reset_count==30]
  data: reset_count local double; reset_input input; reset_state output; run_flag input

== matlab function E55_1030/Function-Call Subsystem2/If Action Subsystem15/MATLAB Function1 ==
  data: SOC input; brake_pressure_f input; brake_pressure_r input; torque_regen_f output; AMKSpeed input; MaxCellVolt input; torque_regen_r output
function [torque_regen_f,torque_regen_r] = regenerate(SOC, brake_pressure_f, brake_pressure_r, AMKSpeed, MaxCellVolt)
% n < 9000rpm时，恒转矩动能回收，n > 9000rpm时，恒功率动能回收
% 效率为1，Ud*Id = T*n
Ud = 500; Id = 12;

Speed1 = 200; % 极低速停止回收
Speed2 = 4000;% 低速保护
Speed3 = 9000;% 恒转矩与恒功率分界线

% 计算最大电磁转矩
if AMKSpeed < Speed1
    T_max = 0;
elseif AMKSpeed < Speed2
    T_max = ((Ud*Id)/(Speed3*pi/30))*(AMKSpeed - 200)/3800;
elseif AMKSpeed < Speed3
    T_max = (Ud*Id)/(Speed3*pi/30);
else
    T_max = (Ud*Id)/(AMKSpeed*pi/30);
end

% SOC系数
if SOC < 30
    factor_T = 1.5;
elseif SOC < 40
    factor_T = -(SOC-30)/20+1.5;
elseif SOC < 60
    factor_T = 1;
elseif SOC < 70
    factor_T = -(SOC-60)*2/30+1;
elseif SOC < 75
    factor_T = 1/3;
elseif SOC < 80
    factor_T = -(SOC-75)/15+1/3;
else 
    factor_T = 0;
end

% 需求电磁转矩
if MaxCellVolt <= 4.2
    T_em_f = factor_T*T_max*max(0, min(1, (brake_pressure_f- 0.5)/2.5));% 限幅为0到1
    T_em_r = factor_T*T_max*max(0, min(1, (brake_pressure_r- 0.5)/2.5));% 限幅为0到1
else
    T_em_f = 0;
    T_em_r = 0;
end

% 归一化并输出
torque_regen_f = -1000*T_em_f/9.8;
torque_regen_r = -1000*T_em_r/9.8;
